simulink model "Hinf_Sem_Incertezas_Realimentacao_an_Com_Atuador"  (R2013b)
settings: Solver=ode45  StartTime=0.0  StopTime=5  RelTol=1e-3
values from neighbouring files (symbols this model uses):
  An = [-1.02   0.905 ... (first row only)    [Incertezas.m]    (also in Main.m; Teste_paper_Robusto_ITA_My_Analisis.m)
  Bn = [ -0.0215 ... (first row only)    [Incertezas.m]    (also in Main.m; Teste_paper_Robusto_ITA_My_Analisis.m)
  Cn = [    0  57.295 ... (first row only)    [Incertezas.m]    (also in Main.m; Teste_paper_Robusto_ITA_My_Analisis.m)
  Dn = [     0 ... (first row only)    [Incertezas.m]    (also in Main.m; Teste_paper_Robusto_ITA_My_Analisis.m)
  k_i = T.Blocks.ki.Value    [Incertezas.m]    (also in comparacao_paper.m)
  k_p = T.Blocks.kp.Value    [Incertezas.m]    (also in comparacao_paper.m)
  k_q = T.Blocks.kq.Value    [Incertezas.m]    (also in comparacao_paper.m)
settings Model: Creator=Eduardo  LastModifiedBy=Eduardo

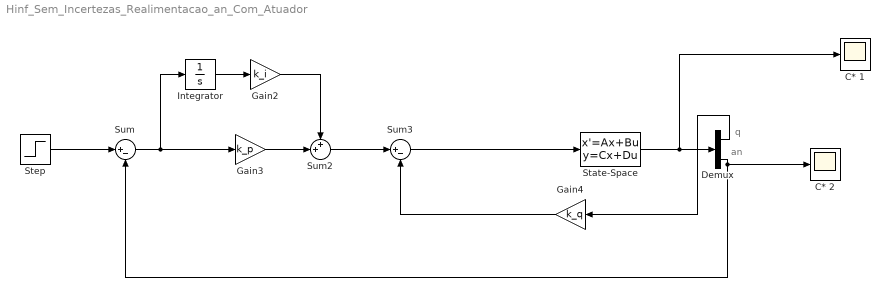
== system Hinf_Sem_Incertezas_Realimentacao_an_Com_Atuador ==
  note: an
  note: q
  C* 1 : Scope
  C* 2 : Scope
  Demux : Demux  Outputs=2
  Gain2 : Gain  Gain=k_i
  Gain3 : Gain  Gain=k_p
  Gain4 : Gain  Gain=k_q
  Integrator : Integrator
  State-Space : StateSpace  A=An  B=Bn  C=Cn  D=Dn  X0=0
  Step : Step  Time=0  SampleTime=0
  Sum : Sum  Inputs=|+-
  Sum2 : Sum  Inputs=++|
  Sum3 : Sum  Inputs=|+-
  wires:
  State-Space/1 -> Demux/1, C* 1/1
  Step/1 -> Sum/1
  Demux/2 -> C* 2/1, Sum/2
  Demux/1 -> Gain4/1
  Sum/1 -> Gain3/1, Integrator/1
  Integrator/1 -> Gain2/1
  Gain2/1 -> Sum2/1
  Gain3/1 -> Sum2/2
  Gain4/1 -> Sum3/2
  Sum2/1 -> Sum3/1
  Sum3/1 -> State-Space/1
